simulink model "singlePhasingFault2023a"  (R2023a)
settings: Solver=VariableStepAuto  StartTime=0.0  StopTime=4  RelTol=1e-3
libraries: spsACVoltageSourceLib x3, spsAsynchronousMachineSIUnitsLib x1, spsGroundLib x1, spsThreePhaseVIMeasurementLib x1, spsdq0toabcLib x1, spspowerguiLib x1
settings Model: Creator=user  LastModifiedBy=admin
settings DataIOCC: ReturnWorkspaceOutputs=off  LoggingToFile=on

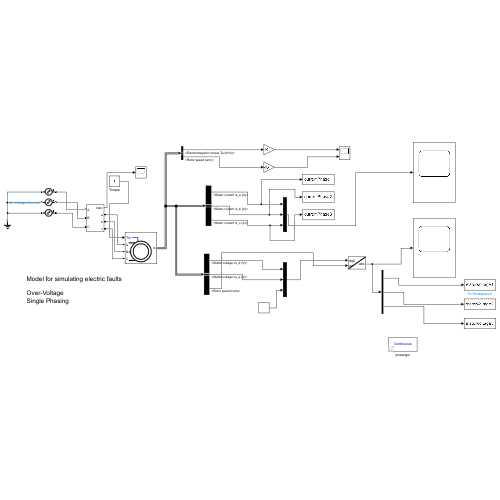
[thumbnail: Simulink's stored preview of the top-level diagram]
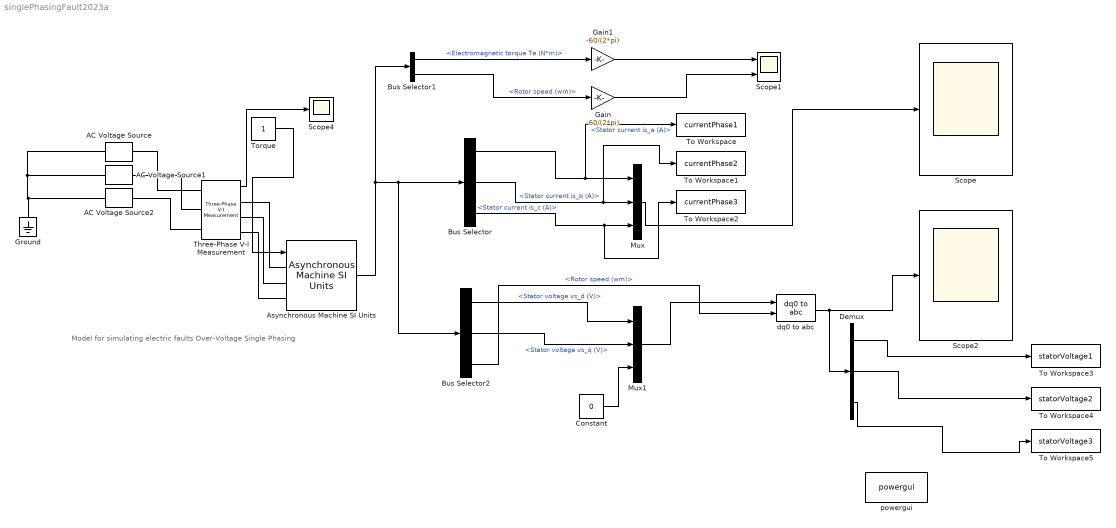
== system singlePhasingFault2023a ==
  note: Model for simulating electric faults
      |
      | Over-Voltage
      | Single Phasing
  AC Voltage Source : spsACVoltageSourceLib/AC Voltage Source  Amplitude=230  Phase=0  Frequency=50  SampleTime=0  Measurements=Voltage  BusType=swing  Pref=10e3  Qref=0  Qmin=-inf  Qmax=+inf
  AC Voltage Source1 : spsACVoltageSourceLib/AC Voltage Source  Amplitude=0  Phase=120  Frequency=50  SampleTime=0  Measurements=None  BusType=swing  Pref=10e3  Qref=0  Qmin=-inf  Qmax=+inf
  AC Voltage Source2 : spsACVoltageSourceLib/AC Voltage Source  Amplitude=230  Phase=-120  Frequency=50  SampleTime=0  Measurements=None  BusType=swing  Pref=10e3  Qref=0  Qmin=-inf  Qmax=+inf
  Asynchronous Machine SI Units : spsAsynchronousMachineSIUnitsLib/Asynchronous Machine SI Units  RotorType=Squirrel-cage  PresetModel="15:  5.4 HP (4KW)   400 V  50Hz 1430 RPM"  MechanicalLoad=Torque Tm  ShowDetailedParameters=on  ReferenceFrame=Stationary  Units=SI  MeasurementBus=off  NominalParameters=[4000 400 50]  VoltageRatio=1  Stator=[1.405 0.005839]  Rotor=[1.395 0.005839]  Cage1=[0.4155 0.002066]  Cage2=[0.4168 0.0003495]  Lm=0.1722  Mechanical=[0.0131 0.002985 2]  PolePairs=2  InitialConditions=[0 0 0 0 0 0 0 0]  SimulateSaturation=off  Saturation=[14.03593122, 27.81365428, 53.79336849, 72.68890987, 97.98006896, 148.6815601, 215.7428561, 302.9841135, 428.7778367 ; 230, 322, 414, 460, 506, 552, 598, 644, 690]  LoadFlowParameters=1492000  TsPowergui=0  TsBlock=-1  IterativeModel=Trapezoidal non iterative  IterativeDiscreteModel=Trapezoidal non iterative  Pmec=1.492e+006
  Bus Selector : BusSelector  OutputSignals=Stator measurements.Stator current is_a (A),Stator measurements.Stator current is_b (A),Stator measurements.Stator current is_c (A)
  Bus Selector1 : BusSelector  OutputSignals=Mechanical.Electromagnetic torque Te (N*m),Mechanical.Rotor speed (wm)
  Bus Selector2 : BusSelector  OutputSignals=Stator measurements.Stator voltage vs_d (V),Stator measurements.Stator voltage vs_q (V),Mechanical.Rotor speed (wm)
  Constant : Constant  Value=0
  Demux : Demux  Outputs=3
  Gain : Gain  Gain=-60/(2*pi)
  Gain1 : Gain  Gain=-60/(2*pi)
  Ground : spsGroundLib/Ground  LConnTagsString=a
  Mux : Mux  Inputs=3
  Mux1 : Mux  Inputs=3
  Scope : Scope
  Scope1 : Scope  NumInputPorts=2
  Scope2 : Scope
  Scope4 : Scope
  Three-Phase V-I Measurement : spsThreePhaseVIMeasurementLib/Three-Phase V-I Measurement  VoltageMeasurement=phase-to-ground  SetLabelV=off  LabelV=Vabc  Vpu=off  VpuLL=off  CurrentMeasurement=no  SetLabelI=off  LabelI=Iabc  Ipu=off  Pbase=100e6  Vbase=500e3  OutputType=Complex  PhasorSimulation=off  PSBequivalent=0
  To Workspace : ToWorkspace  VariableName=currentPhase1  SaveFormat=Timeseries  SampleTime=-1
  To Workspace1 : ToWorkspace  VariableName=currentPhase2  SaveFormat=Timeseries  SampleTime=-1
  To Workspace2 : ToWorkspace  VariableName=currentPhase3  SaveFormat=Timeseries  SampleTime=-1
  To Workspace3 : ToWorkspace  VariableName=statorVoltage1  SaveFormat=Timeseries  SampleTime=-1
  To Workspace4 : ToWorkspace  VariableName=statorVoltage2  SaveFormat=Timeseries  SampleTime=-1
  To Workspace5 : ToWorkspace  VariableName=statorVoltage3  SaveFormat=Timeseries  SampleTime=-1
  Torque : Constant
  dq0 to abc : spsdq0toabcLib/dq0 to abc  Alignment=90 degrees behind phase A axis
  powergui : spspowerguiLib/powergui  Priority=1  SimulationMode=Continuous  SampleTime=50e-6  frequency=60  Iterations=50  frequencyindice=50  Pbase=100e6  ErrMax=1e-4  UnitsV=kV  UnitsW=MW  buscounter=0  FunctionMessages=off  echomessages=off  EnableUseOfTLC=off  CurrentSourceSwitches=off  DisableSnubberDevices=off  DisableRonSwitches=off  DisableVfSwitches=off  DisplayEquations=off  AutomaticDiscreteSolvers=off  SolverType=Tustin/Backward Euler (TBE)  Interpol=off  ExternalGateDelay=off  methode=off  Ts=100  x0status=blocks  SPID=on  SwTol=0  HookPort=off  NonlinearTolerance=1e-4  nMaxIteration=100  ContinueOnMaxIteration=off  RestoreLinks=warning  ResistiveCurrentMeasurement=off  Frange=[0:2:500]  Ylog=off  Xlog=on  ShowGrid=off  save=off  variable=ZData  structure=0  ZoomFFT=off  StartTime=0.0  cycles=1  DisplayStyle=1  fundamental=60  FreqAxis=off  MaxFrequency=1000  frequencyindicesteady=1  RmsSteady=1  display=off
  wires:
  Asynchronous Machine SI Units/1 -> Bus Selector1/1, Bus Selector2/1, Bus Selector/1
  Bus Selector1/2 -> Gain/1  "<Rotor speed (wm)>"
  Gain/1 -> Scope1/2
  Torque/1 -> Asynchronous Machine SI Units/1
  Three-Phase V-I Measurement/1 -> Scope4/1
  Bus Selector1/1 -> Gain1/1  "<Electromagnetic torque Te (N*m)>"
  Gain1/1 -> Scope1/1
  Bus Selector/1 -> Mux/1, To Workspace/1  "<Stator current is_a (A)>"
  Bus Selector/2 -> To Workspace1/1, Mux/2  "<Stator current is_b (A)>"
  Bus Selector/3 -> To Workspace2/1, Mux/3  "<Stator current is_c (A)>"
  Mux/1 -> Scope/1
  Bus Selector2/1 -> Mux1/1  "<Stator voltage vs_d (V)>"
  Bus Selector2/2 -> Mux1/2  "<Stator voltage vs_q (V)>"
  Bus Selector2/3 -> dq0 to abc/2  "<Rotor speed (wm)>"
  Constant/1 -> Mux1/3
  Mux1/1 -> dq0 to abc/1
  dq0 to abc/1 -> Demux/1, Scope2/1
  Demux/1 -> To Workspace3/1
  Demux/3 -> To Workspace5/1
  Demux/2 -> To Workspace4/1
  connections:
  Three-Phase V-I Measurement/RConn1 -- Asynchronous Machine SI Units/LConn1
  Three-Phase V-I Measurement/RConn2 -- Asynchronous Machine SI Units/LConn2
  Three-Phase V-I Measurement/RConn3 -- Asynchronous Machine SI Units/LConn3
  AC Voltage Source/RConn1 -- Three-Phase V-I Measurement/LConn1
  AC Voltage Source1/RConn1 -- Three-Phase V-I Measurement/LConn2
  AC Voltage Source2/RConn1 -- Three-Phase V-I Measurement/LConn3
  Ground/LConn1 -- AC Voltage Source/LConn1 -- AC Voltage Source1/LConn1 -- AC Voltage Source2/LConn1
